simulink model "inlamningregler31"  (R2015a)
settings: Solver=ode45  StartTime=0.0  StopTime=150  RelTol=1e-3
settings Model: Creator=mikpau  LastModifiedBy=mikpau

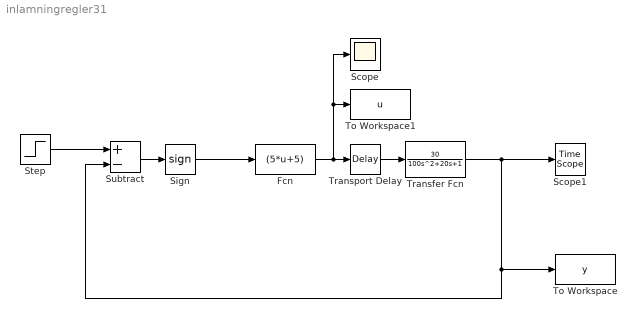
== system inlamningregler31 ==
  Fcn : Fcn  Expr=(5*u+5)
  Scope : Scope
  Scope1 : TimeScope
  Sign : Signum
  Step : Step  After=150  SampleTime=0
  Subtract : Sum  Inputs=+-
  To Workspace : ToWorkspace  VariableName=y  SaveFormat=Timeseries  SampleTime=-1
  To Workspace1 : ToWorkspace  VariableName=u  SaveFormat=Timeseries  SampleTime=-1
  Transfer Fcn : TransferFcn  Numerator=[30]  Denominator=[100 20 1]
  Transport Delay : TransportDelay  DelayTime=10
  wires:
  Transfer Fcn/1 -> Subtract/2, To Workspace/1, Scope1/1
  Subtract/1 -> Sign/1
  Sign/1 -> Fcn/1
  Step/1 -> Subtract/1
  Transport Delay/1 -> Transfer Fcn/1
  Fcn/1 -> Scope/1, To Workspace1/1, Transport Delay/1
